simulink model "ACCsystem"  (R2020a)
settings: Solver=FixedStepAuto  StartTime=0.0  StopTime=T  RelTol=1e-3
values from neighbouring files (symbols this model uses):
  Ts = 0.05    [AdaptiveCruiseControl.m]
  v0_ego = 30    [AdaptiveCruiseControl.m]
  v0_lead = 30    [AdaptiveCruiseControl.m]
  v0_rear = 30    [AdaptiveCruiseControl.m]
  v_set = 100    [AdaptiveCruiseControl.m]
  x0_ego = 20    [AdaptiveCruiseControl.m]
  x0_lead = 80    [AdaptiveCruiseControl.m]
  x0_rear = 14    [AdaptiveCruiseControl.m]
settings Model: Creator=The MathWorks, Inc.  LastModifiedBy=andre
settings DataIOCC: ReturnWorkspaceOutputs=off
settings DebuggingCC: ArithmeticOperatorsInVariantConditions=warning
settings SFSimCC: SimUseLocalCustomCode=off  CustomCodeUndefinedFunction=UseInterfaceOnly
settings RTWCC: RTWUseLocalCustomCode=off
settings CodeAppCC: StateflowObjectComments=on

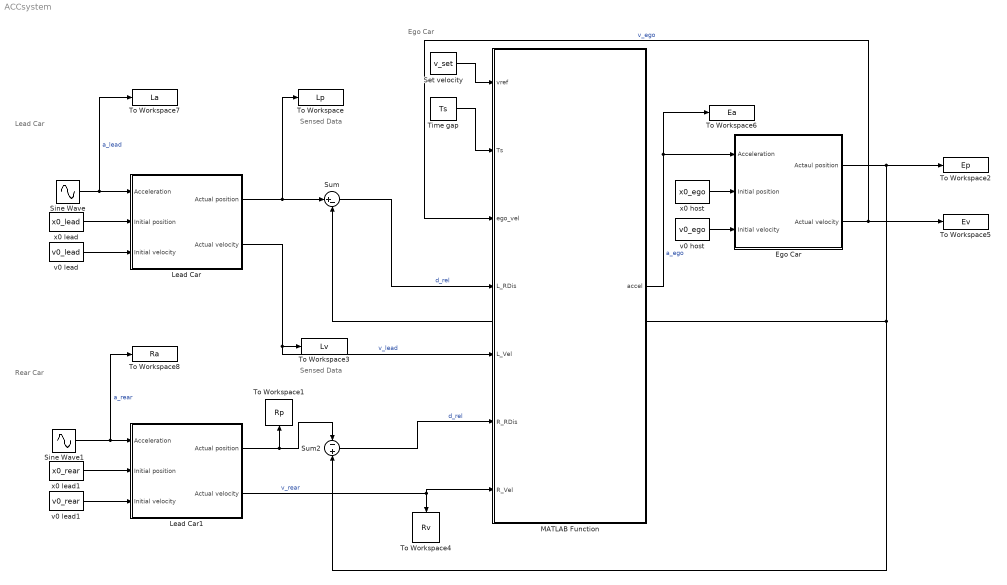
== system ACCsystem ==
  note: Sensed Data
  note: Lead Car
  note: Ego Car
  note: Rear Car
  note: Sensed Data
  Ego Car : Subsystem
  Lead Car : Subsystem
  Lead Car1 : Subsystem
  MATLAB Function : MATLAB Function  TreatAsAtomicUnit=on
  Set velocity : Constant  Value=v_set  SampleTime=Ts
  Sine Wave : Sin  Frequency=0.3  SampleTime=Ts
  Sine Wave1 : Sin  Frequency=0.3  SampleTime=Ts
  Sum : Sum  Inputs=|+-
  Sum2 : Sum  Inputs=-+
  Time gap : Constant  Value=Ts  SampleTime=Ts
  To Workspace : ToWorkspace  VariableName=Lp  SaveFormat=Timeseries  SampleTime=-1
  To Workspace1 : ToWorkspace  VariableName=Rp  SaveFormat=Timeseries  SampleTime=-1
  To Workspace2 : ToWorkspace  VariableName=Ep  SaveFormat=Timeseries  SampleTime=-1
  To Workspace3 : ToWorkspace  VariableName=Lv  SaveFormat=Timeseries  SampleTime=-1
  To Workspace4 : ToWorkspace  VariableName=Rv  SaveFormat=Timeseries  SampleTime=-1
  To Workspace5 : ToWorkspace  VariableName=Ev  SaveFormat=Timeseries  SampleTime=-1
  To Workspace6 : ToWorkspace  VariableName=Ea  SaveFormat=Timeseries  SampleTime=-1
  To Workspace7 : ToWorkspace  VariableName=La  SaveFormat=Timeseries  SampleTime=-1
  To Workspace8 : ToWorkspace  VariableName=Ra  SaveFormat=Timeseries  SampleTime=-1
  v0 host : Constant  Value=v0_ego  SampleTime=Ts
  v0 lead : Constant  Value=v0_lead  SampleTime=Ts
  v0 lead1 : Constant  Value=v0_rear  SampleTime=Ts
  x0 host : Constant  Value=x0_ego  SampleTime=Ts
  x0 lead : Constant  Value=x0_lead  SampleTime=Ts
  x0 lead1 : Constant  Value=x0_rear  SampleTime=Ts
  wires:
  x0 lead/1 -> Lead Car/2(Initial position)
  v0 lead/1 -> Lead Car/3(Initial velocity)
  x0 host/1 -> Ego Car/2(Initial position)
  v0 host/1 -> Ego Car/3(Initial velocity)
  Set velocity/1 -> MATLAB Function/1(vref)
  MATLAB Function/1(accel) -> To Workspace6/1, Ego Car/1(Acceleration)  "a_ego"
  Lead Car/1(Actual position) -> To Workspace/1, Sum/1
  Time gap/1 -> MATLAB Function/2(Ts)
  Sine Wave/1 -> To Workspace7/1, Lead Car/1(Acceleration)  "a_lead"
  Lead Car/2(Actual velocity) -> To Workspace3/1, MATLAB Function/5(L_Vel)  "v_lead"
  Sum/1 -> MATLAB Function/4(L_RDis)  "d_rel"
  v0 lead1/1 -> Lead Car1/3(Initial velocity)
  Sine Wave1/1 -> To Workspace8/1, Lead Car1/1(Acceleration)  "a_rear"
  x0 lead1/1 -> Lead Car1/2(Initial position)
  Lead Car1/2(Actual velocity) -> MATLAB Function/7(R_Vel), To Workspace4/1  "v_rear"
  Ego Car/2(Actual velocity) -> To Workspace5/1, MATLAB Function/3(ego_vel)  "v_ego"
  Sum2/1 -> MATLAB Function/6(R_RDis)  "d_rel"
  Lead Car1/1(Actual position) -> Sum2/1, To Workspace1/1
  Ego Car/1(Actaul position) -> To Workspace2/1, Sum2/2, Sum/2

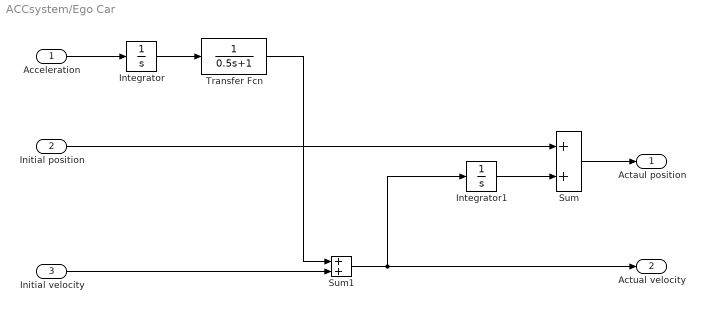
== system ACCsystem/Ego Car ==
  Acceleration : Inport
  Initial position : Inport  Port=2
  Initial velocity : Inport  Port=3
  Integrator : Integrator
  Integrator1 : Integrator
  Sum : Sum
  Sum1 : Sum
  Transfer Fcn : TransferFcn  Denominator=[0.5 1]
  Actaul position : Outport  VectorParamsAs1DForOutWhenUnconnected=off
  Actual velocity : Outport  Port=2  VectorParamsAs1DForOutWhenUnconnected=off
  wires:
  Sum1/1 -> Integrator1/1, Actual velocity/1
  Initial velocity/1 -> Sum1/2
  Sum/1 -> Actaul position/1
  Transfer Fcn/1 -> Sum1/1
  Integrator/1 -> Transfer Fcn/1
  Acceleration/1 -> Integrator/1
  Initial position/1 -> Sum/1
  Integrator1/1 -> Sum/2

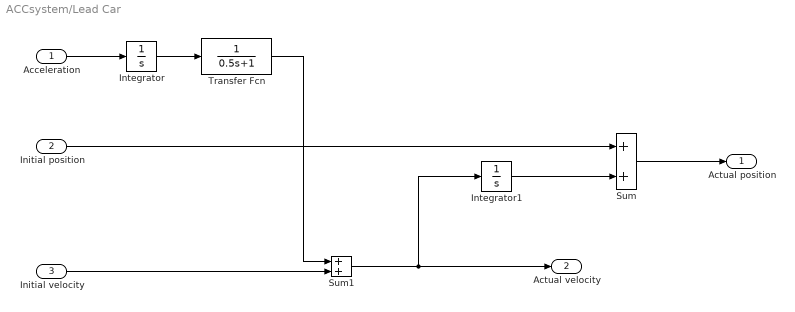
== system ACCsystem/Lead Car ==
  Acceleration : Inport
  Initial position : Inport  Port=2
  Initial velocity : Inport  Port=3
  Integrator : Integrator
  Integrator1 : Integrator
  Sum : Sum
  Sum1 : Sum
  Transfer Fcn : TransferFcn  Denominator=[0.5 1]
  Actual position : Outport  VectorParamsAs1DForOutWhenUnconnected=off
  Actual velocity : Outport  Port=2  VectorParamsAs1DForOutWhenUnconnected=off
  wires:
  Transfer Fcn/1 -> Sum1/1
  Initial velocity/1 -> Sum1/2
  Sum/1 -> Actual position/1
  Integrator/1 -> Transfer Fcn/1
  Sum1/1 -> Integrator1/1, Actual velocity/1
  Acceleration/1 -> Integrator/1
  Initial position/1 -> Sum/1
  Integrator1/1 -> Sum/2

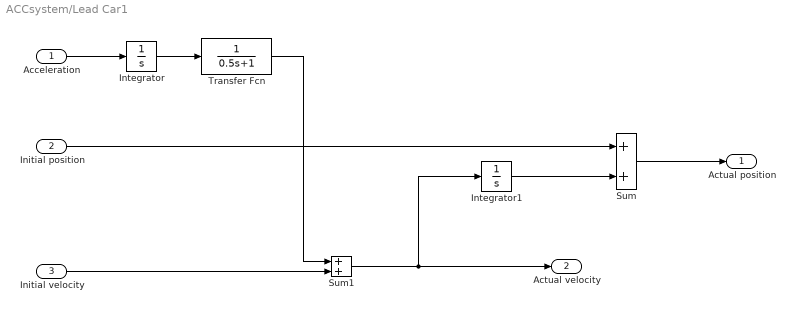
== system ACCsystem/Lead Car1 ==
  Acceleration : Inport
  Initial position : Inport  Port=2
  Initial velocity : Inport  Port=3
  Integrator : Integrator
  Integrator1 : Integrator
  Sum : Sum
  Sum1 : Sum
  Transfer Fcn : TransferFcn  Denominator=[0.5 1]
  Actual position : Outport  VectorParamsAs1DForOutWhenUnconnected=off
  Actual velocity : Outport  Port=2  VectorParamsAs1DForOutWhenUnconnected=off
  wires:
  Transfer Fcn/1 -> Sum1/1
  Initial velocity/1 -> Sum1/2
  Sum/1 -> Actual position/1
  Integrator/1 -> Transfer Fcn/1
  Sum1/1 -> Integrator1/1, Actual velocity/1
  Acceleration/1 -> Integrator/1
  Initial position/1 -> Sum/1
  Integrator1/1 -> Sum/2

== matlab function ACCsystem/MATLAB Function ==
  data: vref input; accel output; Ts input; ego_vel input; L_RDis input; L_Vel input; R_RDis input; R_Vel input
function accel= impPathV2(vref,Ts,ego_vel,L_RDis,L_Vel,R_RDis,R_Vel)
% #1 From a finite acceleration action space select the an acceleration
% #2 Choose and acceleration and check cost function over next 10 sec
a=3.5; %Assume a max acceration of a m/s^2
a_space=-1.2*a:0.01:a;
T=1;    %Projection time of T seconds
t=0:Ts:T;
Mt=repmat(t',1,length(a_space));

eps=10^-6;

%Ego Velocity matrix
V1=t'*a_space+ego_vel;
%TAKE INTO ACCOUNT CHANGE IN DISTANCE FOR Lead and rear
dL=max(L_RDis+(L_Vel-V1).*Mt,eps);
dR=max(R_RDis+(V1-R_Vel).*Mt,eps);

%apply cost function to each velocity
a=0.0005;     %Extends the TTC explosion region
b=7;
Fcost=min(eps,L_Vel-V1).^2 ./ (a*dL.^2);
Rcost=min(eps,V1-R_Vel+0.1).^2 ./ (a*dR.^2);
Scost=b*max(vref-V1,0);

J=Fcost+Rcost+Scost;

%Sum each column to attain cost along trajectory for each acceleration
Js=sum(J,1);
[~,i]=min(Js);
 
accel =a_space(i);
